simulink model "visualize_variables"  (R2023a)
settings: Solver=FixedStepAuto  StartTime=0.0  StopTime=inf  FixedStep=0.1  RelTol=1e-3
libraries: genomix x3
settings Model: Creator=mtognon  LastModifiedBy=swasiela
settings SolverCC: AlgebraicLoopSolver=TrustRegion
settings DataIOCC: ReturnWorkspaceOutputs=off
settings DebuggingCC: UnconnectedInputMsg=warning  UnconnectedOutputMsg=warning  UnconnectedLineMsg=warning  ArithmeticOperatorsInVariantConditions=warning
settings ModelReferenceCC: EnableRefExpFcnMdlSchedulingChecks=on
settings SFSimCC: SimUseLocalCustomCode=off  CustomCodeUndefinedFunction=UseInterfaceOnly
settings RTWCC: RTWUseLocalCustomCode=off

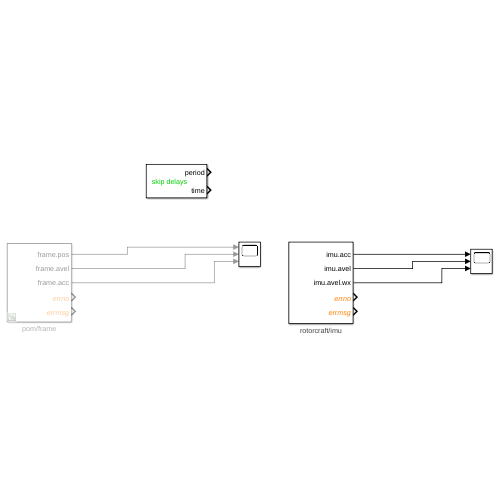
[thumbnail: Simulink's stored preview of the top-level diagram]
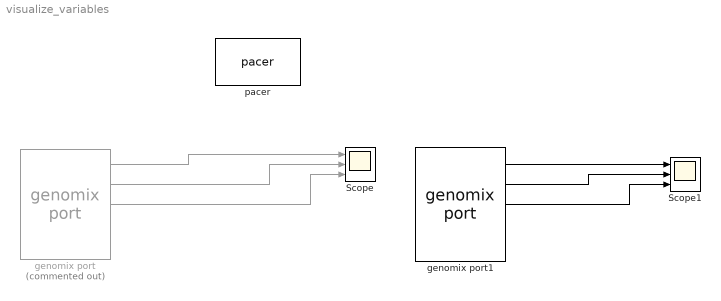
== system visualize_variables ==
  Scope : Scope  NumInputPorts=3
  Scope1 : Scope  NumInputPorts=3
  genomix port : genomix/genomix port  Commented=on  host=erebia-wifi  component=pom  port=frame  subport=robot  sigtype=value  timetype=periodic  period=0.1  siglist="[{\"name\":\"frame.pos\",\"type\":\"value\",\"size\":3},{\"name\":\"frame.avel\",\"type\":\"value\",\"size\":3},{\"name\":\"frame.acc\",\"type\":\"value\",\"size\":3}]"
      settings: AttributesFormatString=pom/frame
  genomix port1 : genomix/genomix port  host=erebia-wifi  component=rotorcraft  port=imu  sigtype=value  timetype=periodic  period=0.1  siglist="[{\"name\":\"imu.acc\",\"type\":\"value\",\"size\":3},{\"name\":\"imu.avel\",\"type\":\"value\",\"size\":3},{\"name\":\"imu.avel.wx\",\"type\":\"value\",\"size\":1}]"
      settings: AttributesFormatString=rotorcraft/imu
  pacer : genomix/pacer  Priority=0  catchup=off
  wires:
  genomix port/1 -> Scope/1
  genomix port1/1 -> Scope1/1
  genomix port/2 -> Scope/2
  genomix port/3 -> Scope/3
  genomix port1/2 -> Scope1/2
  genomix port1/3 -> Scope1/3
